simulink model "Updated_Mode_Selection_3"  (R2022a)
settings: Solver=FixedStepAuto  StartTime=0.0  StopTime=60  FixedStep=1e-3  RelTol=1e-3  EnableMultiTasking=on
undefined symbols (not defined in the file): D10, D11, D12, D13, D2, D3, D4, D5, D6, D7, D8, D9, PTA0, PTA1, PTA2, PTB23, PTB9, PTC2, PTC3, PTC4, PTD0, PTD1, PTD2, PTD3
libraries: frdmk64flib x14
settings Model: ExtModeTrigDuration=5  Creator=ethan  LastModifiedBy=Tamer Rafidi
settings OptimizationCC: EnhancedBackFolding=on  PassReuseOutputArgsAs=Individual arguments  ZeroExternalMemoryAtStartup=off  ZeroInternalMemoryAtStartup=off  MaxStackSize=64  OptimizeBlockOrder=speed  DifferentSizesBufferReuse=on  OptimizationCustomize=off  EfficientTunableParamExpr=on
settings DebuggingCC: ParameterTunabilityLossMsg=error
settings HardwareCC: ProdBitPerPointer=32  ProdBitPerSizeT=32  ProdBitPerPtrDiffT=32  ProdLargestAtomicInteger=Long  ProdLargestAtomicFloat=Double  ProdWordSize=32  ProdHWDeviceType=ARM Compatible->ARM Cortex
settings SFSimCC: MATLABDynamicMemAlloc=off
settings RTWCC: SystemTargetFile=ert.tlc  HardwareBoard=NXP FRDM-K64F  TLCOptions="-aInlineSetEventsForThisBaseRateFcn=TLC_FALSE -aSuppressMultiTaskScheduler=TLC_FALSE  -aRateBasedStepFcn=0"  TemplateMakefile=ert_default_tmf  Toolchain=GNU Tools for ARM Embedded Processors
settings CodeAppCC: ForceParamTrailComments=on  IgnoreCustomStorageClasses=off  OperatorAnnotations=on  SimulinkDataObjDesc=on  SFDataObjDesc=on  InsertBlockDesc=on
settings ERTTargetCC: ExtModeTransport=4  ExtModeMexFile=sendToCommService

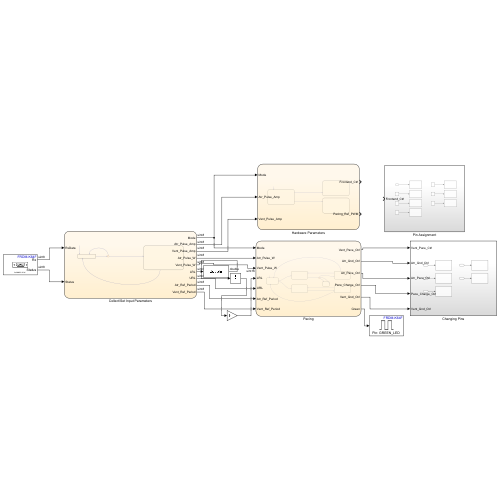
[thumbnail: Simulink's stored preview of the top-level diagram]
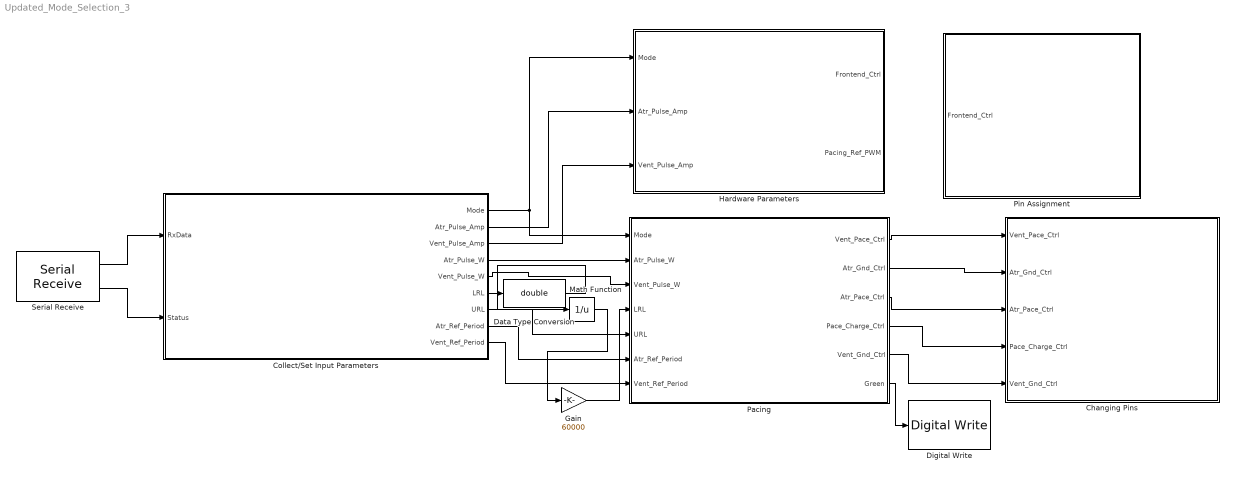
== system Updated_Mode_Selection_3 ==
  Changing Pins : Subsystem
  Collect/Set Input Parameters : Stateflow chart  TreatAsAtomicUnit=on
      settings: PortSchema="{\"entries\":[{\"content\":{\"sides\":[{\"content\":{\"connectorIds\":[\"In1\",\"In2\"]},\"type\":\"ConnectorPlacement.EquallySpacedRectSide\",\"uuid\":\"dc51e4f5-5341-418f-80a9-38d3dc8e9b6e\"},{\"content\":{\"connectorIds\":[\"Out1\",\"Out3\",\"Out6\",\"Out2\",\"Out7\",\"Out9\",\"Out5\",\"Out4\",\"Out8\"],\"side\":\"RIGHT\"},\"type\":\"ConnectorPlacement.EquallySpacedRectSide\",\"uuid\":\"313c6298-b0b7-4ff0-85ba-dbaa1c18177a\"},{\"content\":{\"connectorIds\":[],\"side\":\"TOP\"},\"type\":\"ConnectorPlacement.EquallySpacedRectSide\",\"uuid\":\"6f377806-6de9-4b84-8111-50855010f7f2\"}]},\"type\":\"ConnectorPlacement.EquallySpacedConnector\",\"uuid\":\"8b0403f6-9322-46f9-82a4-778a28822a3d\"}],\"packageUris\":[\"http://schema.mathworks.com/mf0/Connector/R2020b\"],\"version\":\"1.0\"}"
  Data Type Conversion : DataTypeConversion  OutDataTypeStr=double  SaturateOnIntegerOverflow=off  RndMeth=Floor
  Digital Write : frdmk64flib/Digital Write  Whichpin=GREEN_LED
  Gain : Gain  Gain=60000
  Hardware Parameters : Stateflow chart  TreatAsAtomicUnit=on
  Math Function : Math  Operator=reciprocal
  Pacing : Stateflow chart  TreatAsAtomicUnit=on
      settings: PortSchema="{\"entries\":[{\"content\":{\"sides\":[{\"content\":{\"connectorIds\":[\"In7\",\"In1\",\"In3\",\"In5\",\"In2\",\"In6\",\"In4\"]},\"type\":\"ConnectorPlacement.EquallySpacedRectSide\",\"uuid\":\"cbd26b3d-27cb-4744-9a6d-2e29f16e2c2e\"},{\"content\":{\"connectorIds\":[\"Out1\",\"Out2\",\"Out3\",\"Out4\",\"Out5\",\"Out6\"],\"side\":\"RIGHT\"},\"type\":\"ConnectorPlacement.EquallySpacedRectSide\",\"uuid\":\"25c89074-e17e-4898-a31a-c42a3e343a2e\"},{\"content\":{\"connectorIds\":[],\"side\":\"TOP\"},\"type\":\"ConnectorPlacement.EquallySpacedRectSide\",\"uuid\":\"e4014b57-3770-4bf4-bd9b-5c9114757f0a\"}]},\"type\":\"ConnectorPlacement.EquallySpacedConnector\",\"uuid\":\"9ef350bf-8d26-4971-b7d1-0d0774d6b5a5\"}],\"packageUris\":[\"http://schema.mathworks.com/mf0/Connector/R2020b\"],\"version\":\"1.0\"}"
  Pin Assignment : Subsystem
  Serial Receive : frdmk64flib/Serial Receive  SCIModule=0  Baudrate=uint32(9600)  Parity=None  StopBits=1  HardwareFlowControl=None  ByteOrder=LittleEndian  DataType=uint8  DataLength=10  BlockingMode=off  OutputStatus=on  SampleTime=-1
  wires:
  Serial Receive/1 -> Collect/Set Input Parameters/1(RxData)
  Serial Receive/2 -> Collect/Set Input Parameters/2(Status)
  Collect/Set Input Parameters/1(Mode) -> Hardware Parameters/1(Mode), Pacing/7(Mode)
  Collect/Set Input Parameters/3(Atr_Pulse_Amp) -> Hardware Parameters/2(Atr_Pulse_Amp)
  Collect/Set Input Parameters/6(Vent_Pulse_Amp) -> Hardware Parameters/3(Vent_Pulse_Amp)
  Collect/Set Input Parameters/4(Atr_Ref_Period) -> Pacing/6(Atr_Ref_Period)
  Collect/Set Input Parameters/5(URL) -> Pacing/2(URL)
  Collect/Set Input Parameters/9(LRL) -> Data Type Conversion/1
  Collect/Set Input Parameters/8(Vent_Ref_Period) -> Pacing/4(Vent_Ref_Period)
  Collect/Set Input Parameters/2(Atr_Pulse_W) -> Pacing/1(Atr_Pulse_W)
  Pacing/1(Vent_Pace_Ctrl) -> Changing Pins/1(Vent_Pace_Ctrl)
  Pacing/2(Atr_Gnd_Ctrl) -> Changing Pins/2(Atr_Gnd_Ctrl)
  Pacing/3(Atr_Pace_Ctrl) -> Changing Pins/3(Atr_Pace_Ctrl)
  Pacing/4(Pace_Charge_Ctrl) -> Changing Pins/4(Pace_Charge_Ctrl)
  Pacing/5(Vent_Gnd_Ctrl) -> Changing Pins/5(Vent_Gnd_Ctrl)
  Pacing/6(Green) -> Digital Write/1
  Data Type Conversion/1 -> Math Function/1
  Math Function/1 -> Gain/1
  Gain/1 -> Pacing/5(LRL)
  Collect/Set Input Parameters/7(Vent_Pulse_W) -> Pacing/3(Vent_Pulse_W)

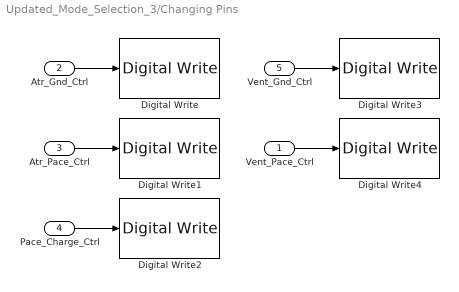
== system Updated_Mode_Selection_3/Changing Pins ==
  Vent_Pace_Ctrl : Inport
  Atr_Gnd_Ctrl : Inport  Port=2
  Atr_Pace_Ctrl : Inport  Port=3
  Pace_Charge_Ctrl : Inport  Port=4
  Vent_Gnd_Ctrl : Inport  Port=5
  Digital Write : frdmk64flib/Digital Write  Whichpin=PTD2 (D11)
  Digital Write1 : frdmk64flib/Digital Write  Whichpin=PTA0 (D8)
  Digital Write2 : frdmk64flib/Digital Write  Whichpin=PTB9 (D2)
  Digital Write3 : frdmk64flib/Digital Write  Whichpin=PTD3 (D12)
  Digital Write4 : frdmk64flib/Digital Write  Whichpin=PTC4 (D9)
  wires:
  Atr_Gnd_Ctrl/1 -> Digital Write/1
  Atr_Pace_Ctrl/1 -> Digital Write1/1
  Pace_Charge_Ctrl/1 -> Digital Write2/1
  Vent_Gnd_Ctrl/1 -> Digital Write3/1
  Vent_Pace_Ctrl/1 -> Digital Write4/1

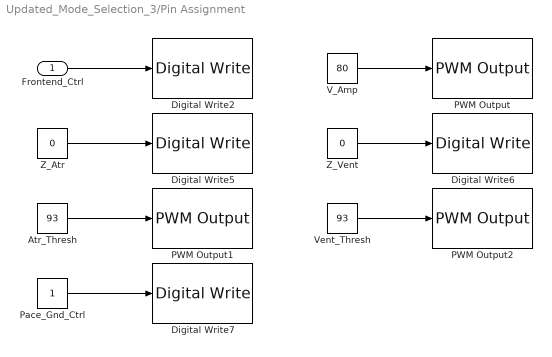
== system Updated_Mode_Selection_3/Pin Assignment ==
  Frontend_Ctrl : Inport
  Atr_Thresh : Constant  Value=93
  Digital Write2 : frdmk64flib/Digital Write  Whichpin=PTD1 (D13)
  Digital Write5 : frdmk64flib/Digital Write  Whichpin=PTB23 (D4)
  Digital Write6 : frdmk64flib/Digital Write  Whichpin=PTC3 (D7)
  Digital Write7 : frdmk64flib/Digital Write  Whichpin=PTD0 (D10)
  PWM Output : frdmk64flib/PWM Output  Whichpin=PTA2 (D5)  InitialFrequency=2000  InitialDutyCycle=0
  PWM Output1 : frdmk64flib/PWM Output  Whichpin=PTC2 (D6)  InitialFrequency=2000  InitialDutyCycle=0
  PWM Output2 : frdmk64flib/PWM Output  Whichpin=PTA1 (D3)  InitialFrequency=2000  InitialDutyCycle=0
  Pace_Gnd_Ctrl : Constant
  V_Amp : Constant  Value=80
  Vent_Thresh : Constant  Value=93
  Z_Atr : Constant  Value=0
  Z_Vent : Constant  Value=0
  wires:
  Frontend_Ctrl/1 -> Digital Write2/1
  V_Amp/1 -> PWM Output/1
  Z_Atr/1 -> Digital Write5/1
  Z_Vent/1 -> Digital Write6/1
  Vent_Thresh/1 -> PWM Output2/1
  Atr_Thresh/1 -> PWM Output1/1
  Pace_Gnd_Ctrl/1 -> Digital Write7/1

== stateflow chart Updated_Mode_Selection_3/Pacing ==
  state VOO_Charge
    entry:
    Vent_Pace_Ctrl = false;
    Vent_Gnd_Ctrl = true;
    Pace_Charge_Ctrl = true;
  state VOO_Discharge
    entry:
    Vent_Pace_Ctrl = true;
    Vent_Gnd_Ctrl = false;
    Pace_Charge_Ctrl = false;
  state Initial_State
    entry:
  state Light
    entry:
    Green = true;
  state AOO_Charge
    entry:
    Green = true;
    Atr_Gnd_Ctrl = false;
    Atr_Pace_Ctrl = false;
  state AOO_Discharge
    entry:
    Green = false;
  VOO_Discharge -> Initial_State [order 1] : [Mode ~= 20]
  VOO_Discharge -> VOO_Charge [order 2] : after(Vent_Pulse_W,msec)
  (junction 66) -> VOO_Discharge [order 2] : [after((LRL)-Vent_Pulse_W,msec)]
  (default) -> Initial_State
  Initial_State -> VOO_Charge [order 1] : [Mode == 20]
  VOO_Charge -> (junction 66)
  Light -> (junction 66)
  (junction 66) -> Light [order 1] : [LRL == 1000]
  Initial_State -> AOO_Charge [order 2] : [Mode == 22]
  AOO_Discharge -> Initial_State [order 1] : [Mode ~= 22]
  AOO_Discharge -> AOO_Charge [order 2] : after(LRL,msec)
  AOO_Charge -> AOO_Discharge : after(LRL,msec)
  data: Atr_Pulse_W input; URL input; Vent_Pulse_W input uint8; Vent_Ref_Period input; LRL input double; Atr_Ref_Period input; Mode input; Vent_Pace_Ctrl output boolean; Atr_Gnd_Ctrl output boolean; Atr_Pace_Ctrl output boolean; Pace_Charge_Ctrl output; Vent_Gnd_Ctrl output; Cur_Mode local; Green output

== stateflow chart Updated_Mode_Selection_3/Hardware Parameters ==
  state Set_Parameters_VOO_VOOR
    entry:
    Pacing_Ref_PWM = (Vent_Pulse_Amp/5)*100;
    Frontend_Ctrl = false;
  state Initialize_Variables
    entry:
    Frontend_Ctrl = false;
  state Set_Parameters_AOO_AOOR
    entry:
    Pacing_Ref_PWM = (Atr_Pulse_Amp/5)*100;
    Frontend_Ctrl = false;
  (default) -> Initialize_Variables
  Initialize_Variables -> Set_Parameters_VOO_VOOR [order 1] : [Mode == 20 || Mode == 5]
  Initialize_Variables -> Set_Parameters_AOO_AOOR [order 2] : [Mode == 2 || Mode == 6]
  data: Mode input; Atr_Pulse_Amp input; Vent_Pulse_Amp input; Frontend_Ctrl output; Pacing_Ref_PWM output uint8

== stateflow chart Updated_Mode_Selection_3/Collect//Set Input Parameters ==
  state Input_Parameters
    entry:
    Mode = RxData(2);
    LRL = RxData(3);
    URL = RxData(4);
    Vent_Pulse_W = RxData(5);
    Atr_Pulse_W = RxData(6);
    Vent_Pulse_Amp = RxData(7);
    Atr_Pulse_Amp = RxData(8);
    Vent_Ref_Period = RxData(9);
    Atr_Ref_Period = RxData(10);
  state Wait_For_Transmission
  (default) -> Wait_For_Transmission
  (junction 16) -> Wait_For_Transmission [order 2]
  Wait_For_Transmission -> (junction 16) : [Status == 0]
  (junction 16) -> Input_Parameters [order 1] : [RxData(1) == hex2dec('10')]
  Input_Parameters -> Wait_For_Transmission
  data: RxData input; Status input; Mode output; Atr_Pulse_W output uint8; Atr_Pulse_Amp output uint8; Atr_Ref_Period output uint8; URL output uint8; Vent_Pulse_Amp output uint8; Vent_Pulse_W output uint8; Vent_Ref_Period output uint8; LRL output uint8
